simulink model "DinamicaDirecta"  (R2019b)
settings: Solver=VariableStepAuto  StartTime=0.0  StopTime=10  RelTol=1e-3
undefined symbols (not defined in the file or in its folder): din_dir
settings Model: Creator=pedro  LastModifiedBy=pedro

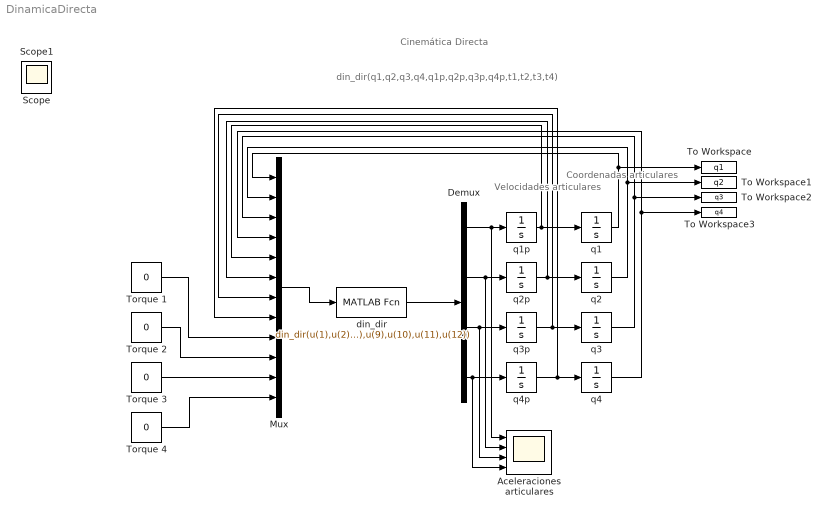
== system DinamicaDirecta ==
  note: Coordenadas
      | articulares
  note: Velocidades
      | articulares
  note: Cinemática Directa
  note: din_dir(q1,q2,q3,q4,q1p,q2p,q3p,q4p,t1,t2,t3,t4)
  "Aceleraciones articulares " : Scope  NumInputPorts=4
  Demux : Demux
  Mux : Mux  Inputs=12
  To Workspace : ToWorkspace  VariableName=q1  SaveFormat=Timeseries  SampleTime=-1
  To Workspace1 : ToWorkspace  VariableName=q2  SaveFormat=Timeseries  SampleTime=-1
  To Workspace2 : ToWorkspace  VariableName=q3  SaveFormat=Timeseries  SampleTime=-1
  To Workspace3 : ToWorkspace  VariableName=q4  SaveFormat=Timeseries  SampleTime=-1
  "Torque 1 " : Constant  Value=0
  Torque 2 : Constant  Value=0
  Torque 3 : Constant  Value=0
  Torque 4 : Constant  Value=0
  din_dir : MATLABFcn  MATLABFcn=din_dir(u(1),u(2),u(3),u(4),u(5),u(6),u(7),u(8),u(9),u(10),u(11),u(12))  OutputDimensions=4
  q{1..4} (4 alike) : Integrator
  q1p : Integrator
  q2p : Integrator
  q3p : Integrator
  q4p : Integrator
  Scope : Scope
  Scope1 : Scope
  wires:
  din_dir/1 -> Demux/1
  Demux/1 -> "Aceleraciones articulares "/1, q1p/1
  Demux/4 -> "Aceleraciones articulares "/4, q4p/1
  Demux/2 -> "Aceleraciones articulares "/2, q2p/1
  Demux/3 -> "Aceleraciones articulares "/3, q3p/1
  q2p/1 -> Mux/6, q2/1
  q4p/1 -> Mux/8, q4/1
  q1p/1 -> Mux/5, q1/1
  q3p/1 -> Mux/7, q3/1
  Mux/1 -> din_dir/1
  q1/1 -> Mux/1, To Workspace/1
  q2/1 -> Mux/2, To Workspace1/1
  q3/1 -> To Workspace2/1, Mux/3
  q4/1 -> To Workspace3/1, Mux/4
  Torque 4/1 -> Mux/12
  Torque 3/1 -> Mux/11
  Torque 2/1 -> Mux/10
  "Torque 1 "/1 -> Mux/9
